simulink model "Quadcopter_Model"  (R2026a)
settings: Solver=FixedStepAuto  StopTime=T  FixedStep=Ts
values from neighbouring files (symbols this model uses):
  a = L/sqrt(2)    [Quadcopter_Commands.m]
  Drag = -0.1    [Quadcopter_Commands.m]
  g = 9.81    [Quadcopter_Commands.m]
  Hover_FeedForward = sqrt((M*g)/(4*Kf))    [Quadcopter_Commands.m]
  Ix = 6*10^(-5)    (= 6e-05)    [Quadcopter_Commands.m]
  Iy = 6*10^(-5)    (= 6e-05)    [Quadcopter_Commands.m]
  Iz = 1.2*10^(-4)    (= 0.00012)    [Quadcopter_Commands.m]
  Kf = 3*10^(-7)    (= 3e-07)    [Quadcopter_Commands.m]
  Km = 3*10^(-9)    (= 3e-09)    [Quadcopter_Commands.m]
  M = 0.07    [Quadcopter_Commands.m]
  Ts = 0.001    [Quadcopter_Commands.m]
undefined symbols (not defined in the file or in its folder): dspblkCoreblockFVToolHelper, gcbh
libraries: simulink x9, matrix_library x5
settings Model: Creator=marco91  LastModifiedBy=marco91
settings OptimizationCC: DefaultUnderspecifiedDataType=single  OptimizeBlockIOStorage=off  BufferReuse=off  OptimizeDataStoreBuffers=off  BusAssignmentInplaceUpdate=off
settings DebuggingCC: ParamPrecisionLossAbsoluteDiffThreshold=0  ParamPrecisionLossRelativeDiffThreshold=0
settings RTWCC: GenCodeOnly=on  GenerateReport=on  BuildConfiguration=Debug  LaunchReport=on
settings CodeAppCC: MATLABSourceComments=on  EnableCustomComments=on
settings GRTTargetCC: MultiInstanceErrorCode=Warning  CombineSignalStateStructs=on  SupportVariableSizeSignals=on

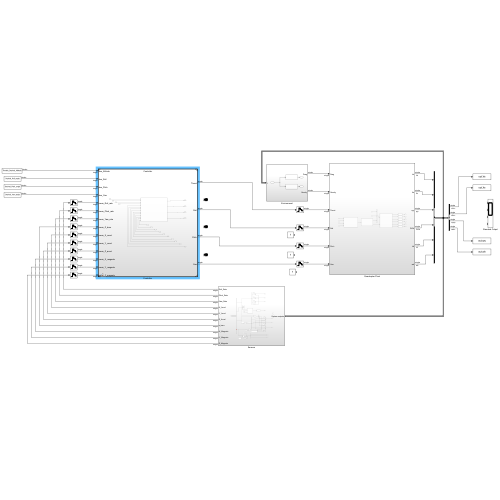
[thumbnail: Simulink's stored preview of the top-level diagram]
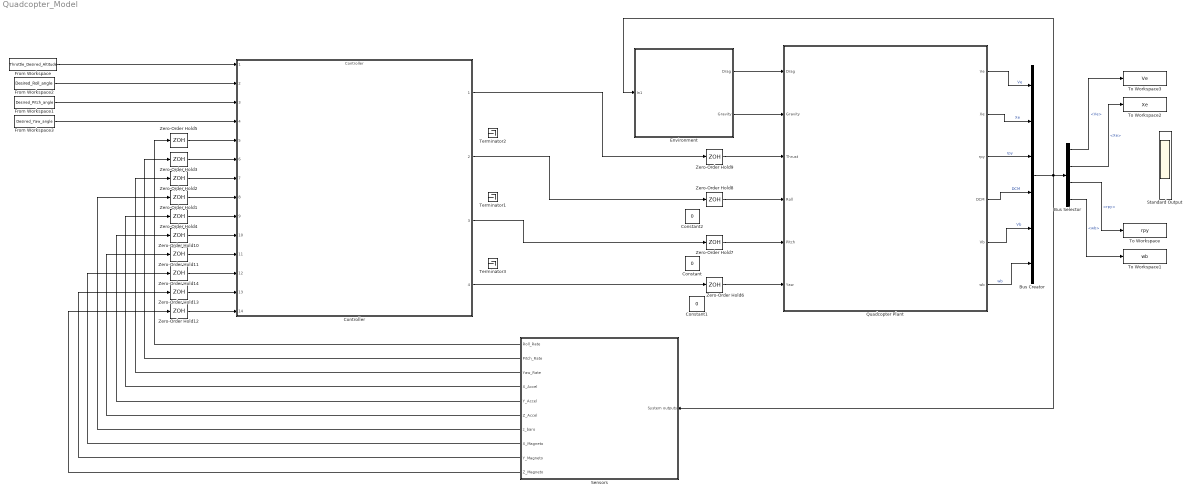
== system Quadcopter_Model ==
  Bus Creator : BusCreator  Inputs=6
  Bus Selector : BusSelector  OutputSignals=Ve,Xe,rpy,wb
  Constant : Constant  Value=0  OutDataTypeStr=single
  Constant1 : Constant  Value=0  OutDataTypeStr=single
  Constant2 : Constant  Value=0  OutDataTypeStr=single
  Controller : ModelReference  ModelNameDialog=Controller  SimulationMode=Normal  ModelReferenceVersion=2.455
  Environment : Subsystem
  From Workspace : FromWorkspace  VariableName=Throttle_Desired_Altitude  SampleTime=Ts
  From Workspace1 : FromWorkspace  VariableName=Desired_Pitch_angle  SampleTime=Ts
  From Workspace2 : FromWorkspace  VariableName=Desired_Roll_angle  SampleTime=Ts
  From Workspace3 : FromWorkspace  VariableName=Desired_Yaw_angle  SampleTime=Ts
  Quadcopter Plant : Subsystem
  Sensors : Subsystem
  Standard Output : Scope  NumInputPorts=4
      settings: ActiveDisplayYMinimum=-2.7234359681606293  ActiveDisplayYMaximum=4.365431159734726
  Terminator1 : Terminator
  Terminator2 : Terminator
  Terminator3 : Terminator
  To Workspace : ToWorkspace  VariableName=rpy  SaveFormat=Timeseries  SampleTime=Ts
  To Workspace1 : ToWorkspace  VariableName=wb  SaveFormat=Timeseries  SampleTime=Ts
  To Workspace2 : ToWorkspace  VariableName=Xe  SaveFormat=Timeseries  SampleTime=Ts
  To Workspace3 : ToWorkspace  VariableName=Ve  SaveFormat=Timeseries  SampleTime=Ts
  Zero-Order Hold1 : ZeroOrderHold  SampleTime=50*Ts
  Zero-Order Hold{2..5,10..11} (6 alike) : ZeroOrderHold  SampleTime=2*Ts
  Zero-Order Hold12 : ZeroOrderHold  SampleTime=10*Ts
  Zero-Order Hold13 : ZeroOrderHold  SampleTime=10*Ts
  Zero-Order Hold14 : ZeroOrderHold  SampleTime=10*Ts
  Zero-Order Hold{6..9} (4 alike) : ZeroOrderHold  SampleTime=Ts
  wires:
  Bus Creator/1 -> Environment/1(In1), Bus Selector/1, Sensors/1(System outputs)
  Bus Selector/1 -> To Workspace3/1  "<Ve>"
  Bus Selector/2 -> To Workspace2/1  "<Xe>"
  Bus Selector/3 -> To Workspace/1  "<rpy>"
  Bus Selector/4 -> To Workspace1/1  "<wb>"
  Quadcopter Plant/1(Ve) -> Bus Creator/1  "Ve"
  Quadcopter Plant/2(Xe) -> Bus Creator/2  "Xe"
  Quadcopter Plant/3(rpy) -> Bus Creator/3  "rpy"
  Quadcopter Plant/4(DCM) -> Bus Creator/4  "DCM"
  Quadcopter Plant/5(Vb) -> Bus Creator/5  "Vb"
  Quadcopter Plant/6(wb) -> Bus Creator/6  "wb"
  From Workspace/1 -> Controller/1
  From Workspace2/1 -> Controller/2
  From Workspace1/1 -> Controller/3
  From Workspace3/1 -> Controller/4
  Zero-Order Hold4/1 -> Controller/9
  Zero-Order Hold5/1 -> Controller/5
  Zero-Order Hold3/1 -> Controller/6
  Zero-Order Hold2/1 -> Controller/7
  Zero-Order Hold1/1 -> Controller/8
  Sensors/1(Roll_Rate) -> Zero-Order Hold5/1
  Sensors/2(Pitch_Rate) -> Zero-Order Hold3/1
  Sensors/3(Yaw_Rate) -> Zero-Order Hold2/1
  Sensors/4(X_Accel) -> Zero-Order Hold4/1
  Sensors/5(Y_Accel) -> Zero-Order Hold10/1
  Sensors/6(Z_Accel) -> Zero-Order Hold11/1
  Zero-Order Hold10/1 -> Controller/10
  Zero-Order Hold11/1 -> Controller/11
  Zero-Order Hold12/1 -> Controller/14
  Zero-Order Hold13/1 -> Controller/13
  Zero-Order Hold14/1 -> Controller/12
  Sensors/7(z_baro) -> Zero-Order Hold1/1
  Sensors/8(X_Magneto) -> Zero-Order Hold14/1
  Sensors/9(Y_Magneto) -> Zero-Order Hold13/1
  Sensors/10(Z_Magneto) -> Zero-Order Hold12/1
  Environment/1(Drag) -> Quadcopter Plant/1(Drag)
  Environment/2(Gravity) -> Quadcopter Plant/2(Gravity)
  Zero-Order Hold9/1 -> Quadcopter Plant/3(Thrust)
  Controller/1 -> Zero-Order Hold9/1
  Zero-Order Hold6/1 -> Quadcopter Plant/6(Yaw)
  Controller/4 -> Zero-Order Hold6/1
  Zero-Order Hold7/1 -> Quadcopter Plant/5(Pitch)
  Zero-Order Hold8/1 -> Quadcopter Plant/4(Roll)
  Controller/3 -> Zero-Order Hold7/1
  Controller/2 -> Zero-Order Hold8/1

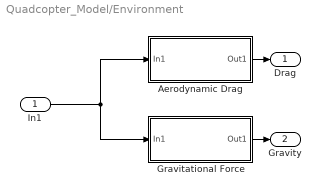
== system Quadcopter_Model/Environment ==
  In1 : Inport  OutDataTypeStr=single
  Aerodynamic Drag : Subsystem
  Gravitational Force : Subsystem
  Drag : Outport
  Gravity : Outport  Port=2
  wires:
  Gravitational Force/1(Out1) -> Gravity/1
  Aerodynamic Drag/1(Out1) -> Drag/1
  In1/1 -> Gravitational Force/1(In1), Aerodynamic Drag/1(In1)

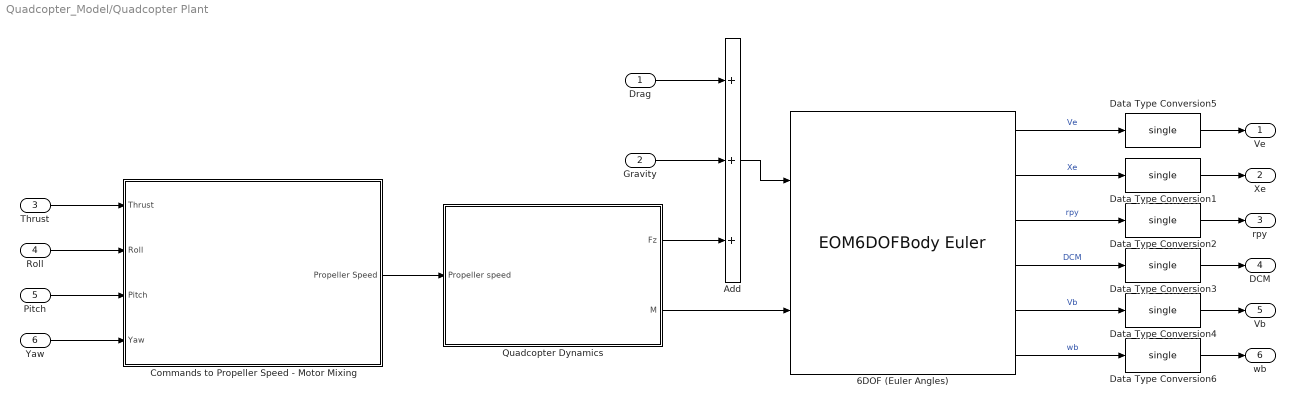
== system Quadcopter_Model/Quadcopter Plant ==
  Drag : Inport  OutDataTypeStr=single
  Gravity : Inport  Port=2  OutDataTypeStr=single
  Thrust : Inport  Port=3  OutDataTypeStr=single
  Roll : Inport  Port=4  OutDataTypeStr=single
  Pitch : Inport  Port=5  OutDataTypeStr=single
  Yaw : Inport  Port=6  OutDataTypeStr=single
  6DOF (Euler Angles) : EOM6DOFBodyEuler  mass_0=M  inertia=[Ix, 0, 0; 0, Iy, 0; 0, 0, Iz]
  Add : Sum  Inputs=+++  OutDataTypeStr=double
  "Commands to Propeller Speed - Motor Mixing " : Subsystem
  Data Type Conversion{1..6} (6 alike) : DataTypeConversion  OutDataTypeStr=single  SaturateOnIntegerOverflow=off  RndMeth=Floor
  Quadcopter Dynamics : Subsystem
  Ve : Outport  OutDataTypeStr=single
  Xe : Outport  Port=2  OutDataTypeStr=single
  rpy : Outport  Port=3  OutDataTypeStr=single
  DCM : Outport  Port=4  OutDataTypeStr=single
  Vb : Outport  Port=5  OutDataTypeStr=single
  wb : Outport  Port=6  OutDataTypeStr=single
  wires:
  "Commands to Propeller Speed - Motor Mixing "/1(Propeller Speed) -> Quadcopter Dynamics/1(Propeller speed)
  Quadcopter Dynamics/1(Fz) -> Add/3
  Quadcopter Dynamics/2(M) -> 6DOF (Euler Angles)/2
  6DOF (Euler Angles)/2 -> Data Type Conversion1/1  "Xe"
  Pitch/1 -> "Commands to Propeller Speed - Motor Mixing "/3(Pitch)
  Add/1 -> 6DOF (Euler Angles)/1
  6DOF (Euler Angles)/5 -> Data Type Conversion4/1  "Vb"
  Thrust/1 -> "Commands to Propeller Speed - Motor Mixing "/1(Thrust)
  6DOF (Euler Angles)/3 -> Data Type Conversion2/1  "rpy"
  6DOF (Euler Angles)/4 -> Data Type Conversion3/1  "DCM"
  Gravity/1 -> Add/2
  6DOF (Euler Angles)/1 -> Data Type Conversion5/1  "Ve"
  6DOF (Euler Angles)/6 -> Data Type Conversion6/1  "wb"
  Drag/1 -> Add/1
  Yaw/1 -> "Commands to Propeller Speed - Motor Mixing "/4(Yaw)
  Roll/1 -> "Commands to Propeller Speed - Motor Mixing "/2(Roll)
  Data Type Conversion6/1 -> wb/1
  Data Type Conversion4/1 -> Vb/1
  Data Type Conversion3/1 -> DCM/1
  Data Type Conversion2/1 -> rpy/1
  Data Type Conversion1/1 -> Xe/1
  Data Type Conversion5/1 -> Ve/1

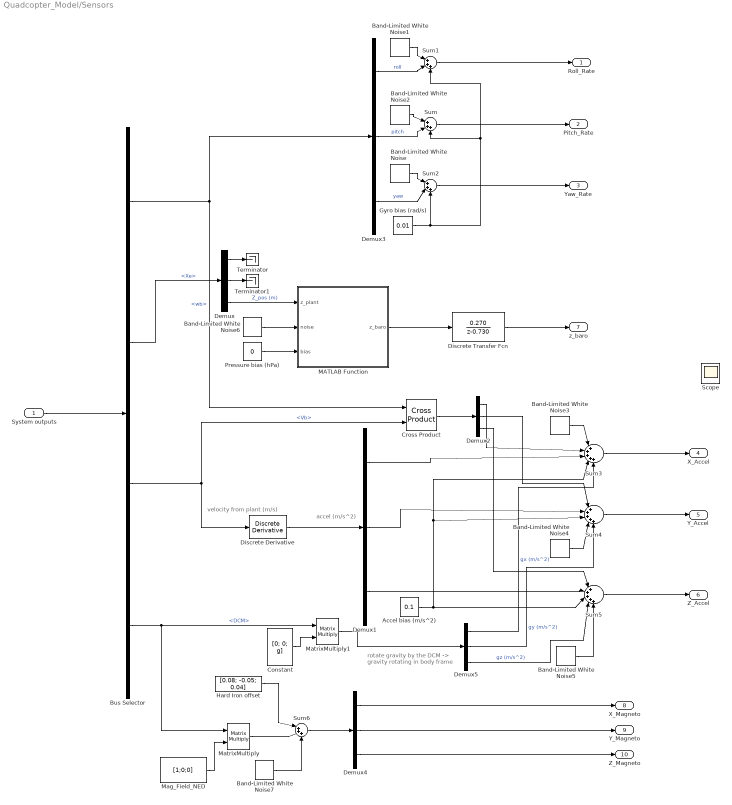
== system Quadcopter_Model/Sensors ==
  note: rotate gravity by the DCM
      | -> gravity rotating in body frame
  note: accel (m/s^2)
  note: velocity from
      | plant (m/s)
  System outputs : Inport
  Accel bias (m/s^2) : Constant  Value=0.1  OutDataTypeStr=single
  Band-Limited White Noise : simulink/Sources/Band-Limited White Noise  Cov=4e-9  Ts=Ts  seed=[23341]
  Band-Limited White Noise1 : simulink/Sources/Band-Limited White Noise  Cov=4e-9  Ts=Ts  seed=[23342]
  Band-Limited White Noise2 : simulink/Sources/Band-Limited White Noise  Cov=4e-9  Ts=Ts  seed=[23343]
  Band-Limited White Noise3 : simulink/Sources/Band-Limited White Noise  Cov=4e-7  Ts=Ts  seed=[23342]
  Band-Limited White Noise4 : simulink/Sources/Band-Limited White Noise  Cov=4e-7  Ts=Ts  seed=[23343]
  Band-Limited White Noise5 : simulink/Sources/Band-Limited White Noise  Cov=4e-7  Ts=Ts  seed=[23341]
  Band-Limited White Noise6 : simulink/Sources/Band-Limited White Noise  Cov=4e-7  Ts=Ts  seed=[23341]
  Band-Limited White Noise7 : simulink/Sources/Band-Limited White Noise  Cov=4e-7  Ts=Ts  seed=[23341]
  Bus Selector : BusSelector  OutputSignals=wb,Xe,Vb,DCM
  Constant : Constant  Value=[0; 0; g]  VectorParams1D=off
  Cross Product : matrix_library/Cross Product
  Demux{,1..5} (6 alike) : Demux  Outputs=3
  Discrete Transfer Fcn : DiscreteTransferFcn  LoadFcn=dspblkCoreblockFVToolHelper(gcbh,'load');  Numerator=[0.270]  Denominator="[1  -0.730]"
      settings: CopyFcn=dspblkCoreblockFVToolHelper(gcbh,'copy');  DeleteFcn=dspblkCoreblockFVToolHelper(gcbh,'close');  ModelCloseFcn=dspblkCoreblockFVToolHelper(gcbh,'close');  PreSaveFcn=dspblkCoreblockFVToolHelper(gcbh,'presave');  PostSaveFcn=dspblkCoreblockFVToolHelper(gcbh,'postsave');  CloseFcn=dspblkCoreblockFVToolHelper(gcbh,'close');
  Discrete Derivative : simulink/Discrete/Discrete Derivative  gainval=1.0  ICPrevScaledInput=0.0  OutMin=[]  OutMax=[]  OutDataTypeStr=single  OutputDataTypeScalingMode=single  OutDataType=fixdt(1, 16)  OutScaling=2^-10  DoSatur=off
  Gyro bias (rad/s) : Constant  Value=0.01  OutDataTypeStr=single
  Hard Iron offset : Constant  Value=[0.08; -0.05; 0.04]  VectorParams1D=off  OutDataTypeStr=single
  MATLAB Function : MATLAB Function  TreatAsAtomicUnit=on
  Mag_Field_NED : Constant  Value=[1;0;0]  VectorParams1D=off
  MatrixMultiply : Product  Multiplication=Matrix(*)
  MatrixMultiply1 : Product  Multiplication=Matrix(*)
  Pressure bias (hPa) : Constant  Value=0  OutDataTypeStr=single
  Scope : Scope
      settings: ActiveDisplayYMinimum=-1  ActiveDisplayYMaximum=1
  Sum{,1..2,6} (4 alike) : Sum  Inputs=|+++  OutDataTypeStr=single
  Sum3 : Sum  Inputs=|+++++  OutDataTypeStr=single
  Sum4 : Sum  Inputs=|+++++  OutDataTypeStr=single
  Sum5 : Sum  Inputs=|+++++  OutDataTypeStr=single
  Terminator : Terminator
  Terminator1 : Terminator
  Roll_Rate : Outport  OutDataTypeStr=single
  Pitch_Rate : Outport  Port=2  OutDataTypeStr=single
  Yaw_Rate : Outport  Port=3  OutDataTypeStr=single
  X_Accel : Outport  Port=4  OutDataTypeStr=single
  Y_Accel : Outport  Port=5  OutDataTypeStr=single
  Z_Accel : Outport  Port=6  OutDataTypeStr=single
  z_baro : Outport  Port=7  OutDataTypeStr=single
  X_Magneto : Outport  Port=8  OutDataTypeStr=single
  Y_Magneto : Outport  Port=9  OutDataTypeStr=single
  Z_Magneto : Outport  Port=10  OutDataTypeStr=single
  wires:
  System outputs/1 -> Bus Selector/1
  Bus Selector/1 -> Cross Product/1, Demux3/1  "<wb>"
  Sum2/1 -> Yaw_Rate/1
  Sum1/1 -> Roll_Rate/1
  Sum/1 -> Pitch_Rate/1
  Demux3/1 -> Sum1/2  "roll"
  Band-Limited White Noise1/1 -> Sum1/1
  Demux3/3 -> Sum2/2  "yaw"
  Demux3/2 -> Sum/2  "pitch"
  Band-Limited White Noise2/1 -> Sum/1
  Band-Limited White Noise/1 -> Sum2/1
  Gyro bias (rad/s)/1 -> Sum1/3, Sum/3, Sum2/3
  Demux1/1 -> Sum3/3
  Demux1/2 -> Sum4/2
  Demux1/3 -> Sum5/2
  Band-Limited White Noise3/1 -> Sum3/1
  Accel bias (m/s^2)/1 -> Sum3/4, Sum4/3, Sum5/3
  Sum4/1 -> Y_Accel/1
  Sum3/1 -> X_Accel/1
  Bus Selector/2 -> Demux/1  "<Xe>"
  Demux/1 -> Terminator/1
  Demux/2 -> Terminator1/1
  Bus Selector/3 -> Discrete Derivative/1, Cross Product/2  "<Vb>"
  Cross Product/1 -> Demux2/1
  Demux2/3 -> Sum5/1
  Demux2/1 -> Sum3/2
  Band-Limited White Noise5/1 -> Sum5/5
  Band-Limited White Noise4/1 -> Sum4/4
  Demux2/2 -> Sum4/1
  Demux/3 -> MATLAB Function/1(z_plant)  "Z_pos (m)"
  Pressure bias (hPa)/1 -> MATLAB Function/3(bias)
  Band-Limited White Noise6/1 -> MATLAB Function/2(noise)
  Mag_Field_NED/1 -> MatrixMultiply/2
  Bus Selector/4 -> MatrixMultiply/1, MatrixMultiply1/1  "<DCM>"
  MatrixMultiply/1 -> Sum6/2
  Band-Limited White Noise7/1 -> Sum6/3
  Hard Iron offset/1 -> Sum6/1
  Sum6/1 -> Demux4/1
  Demux4/1 -> X_Magneto/1
  Demux4/2 -> Y_Magneto/1
  Demux4/3 -> Z_Magneto/1
  Discrete Derivative/1 -> Demux1/1
  Sum5/1 -> Z_Accel/1
  MATLAB Function/1(z_baro) -> Discrete Transfer Fcn/1
  Discrete Transfer Fcn/1 -> z_baro/1
  MatrixMultiply1/1 -> Demux5/1
  Demux5/1 -> Sum3/5  "gx (m/s^2)"
  Demux5/3 -> Sum5/4  "gz (m/s^2)"
  Demux5/2 -> Sum4/5  "gy (m/s^2)"
  Constant/1 -> MatrixMultiply1/2

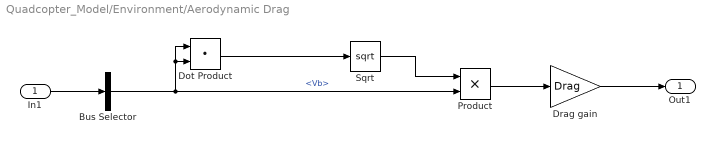
== system Quadcopter_Model/Environment/Aerodynamic Drag ==
  In1 : Inport  OutDataTypeStr=single
  Bus Selector : BusSelector  OutputSignals=Vb
  Dot Product : DotProduct  OutDataTypeStr=single
  Drag gain : Gain  Gain=Drag  OutDataTypeStr=single
  Product : Product  OutDataTypeStr=single
  Sqrt : Sqrt  OutDataTypeStr=single  IntermediateResultsDataTypeStr=single
  Out1 : Outport
  wires:
  Drag gain/1 -> Out1/1
  Product/1 -> Drag gain/1
  Sqrt/1 -> Product/1
  Bus Selector/1 -> Dot Product/1, Dot Product/2, Product/2  "<Vb>"
  In1/1 -> Bus Selector/1
  Dot Product/1 -> Sqrt/1

== system Quadcopter_Model/Environment/Gravitational Force ==
  note: (Gravitational) Force given by the gravitational acceleration multiplied by the mass
  In1 : Inport  OutDataTypeStr=single
  Gravitational Acceleration : Subsystem
  Mass [Kg] : Gain  Gain=M
  Out1 : Outport
  wires:
  In1/1 -> Gravitational Acceleration/1(In1)
  Gravitational Acceleration/1(Out1) -> Mass [Kg]/1
  Mass [Kg]/1 -> Out1/1

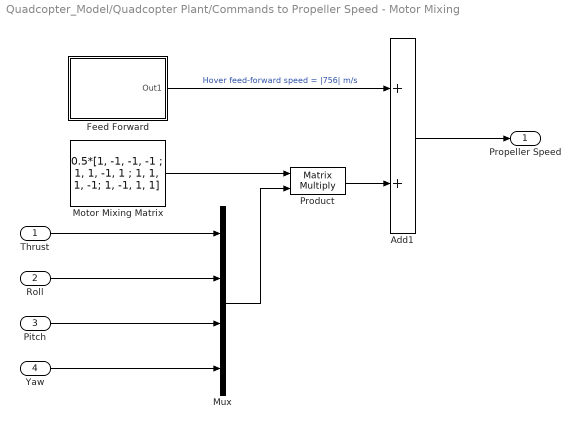
== system Quadcopter_Model/Quadcopter Plant/Commands to Propeller Speed - Motor Mixing  ==
  Thrust : Inport
  Roll : Inport  Port=2  OutDataTypeStr=single
  Pitch : Inport  Port=3  OutDataTypeStr=single
  Yaw : Inport  Port=4  OutDataTypeStr=single
  Add1 : Sum
  Feed Forward : Subsystem
  Motor Mixing Matrix : Constant  Value="0.5*[1, -1, -1, -1 ; 1, 1, -1, 1 ;   1, 1, 1, -1;  1, -1, 1, 1]"  VectorParams1D=off  OutDataTypeStr=single
  Mux : Mux
  Product : Product  Multiplication=Matrix(*)  OutDataTypeStr=single
  Propeller Speed : Outport  OutDataTypeStr=single
  wires:
  Feed Forward/1(Out1) -> Add1/1  "Hover feed-forward speed = |756| m/s"
  Mux/1 -> Product/2
  Pitch/1 -> Mux/3
  Product/1 -> Add1/2
  Roll/1 -> Mux/2
  Motor Mixing Matrix/1 -> Product/1
  Yaw/1 -> Mux/4
  Add1/1 -> Propeller Speed/1
  Thrust/1 -> Mux/1

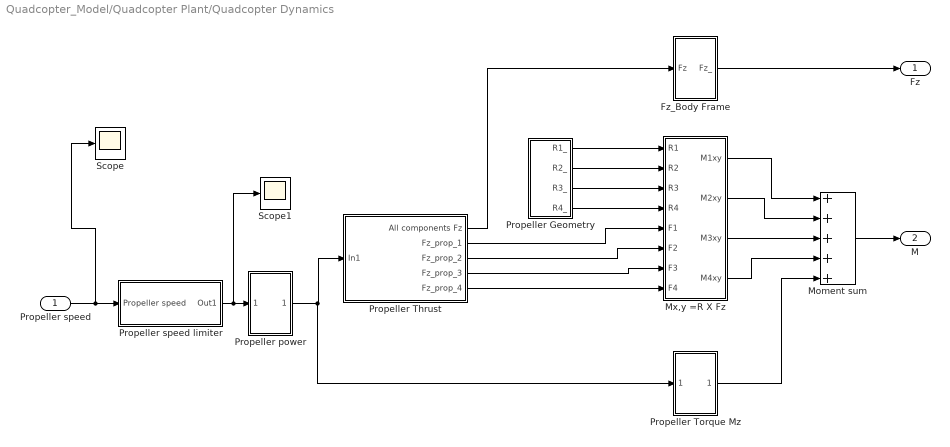
== system Quadcopter_Model/Quadcopter Plant/Quadcopter Dynamics ==
  Propeller speed : Inport  OutDataTypeStr=single
  Fz_Body Frame : Subsystem
  Moment sum : Sum  Inputs=+++++  OutDataTypeStr=double
  Mx,y =R X Fz : Subsystem
  Propeller Geometry : Subsystem
  Propeller Thrust : Subsystem
  Propeller Torque Mz : Subsystem
  Propeller power : Subsystem
  Propeller speed limiter : Subsystem
  Scope : Scope
      settings: ActiveDisplayYMinimum=-967.50824737548828  ActiveDisplayYMaximum=-720.62401580810547  DataLoggingVariableName=ScopeData4
  Scope1 : Scope
      settings: ActiveDisplayYMinimum=-967.50824737548828  ActiveDisplayYMaximum=-720.62401580810547  DataLoggingVariableName=ScopeData2
  Fz : Outport  OutDataTypeStr=single
  M : Outport  Port=2  OutDataTypeStr=double
  wires:
  Propeller speed/1 -> Scope/1, Propeller speed limiter/1(Propeller speed)
  Propeller speed limiter/1(Out1) -> Scope1/1, Propeller power/1(In1)
  Propeller power/1(Out1) -> Propeller Torque Mz/1(In1), Propeller Thrust/1(In1)
  Propeller Thrust/1(All components Fz) -> Fz_Body Frame/1(Fz)
  Propeller Thrust/2(Fz_prop_1) -> Mx,y =R X Fz/5(F1)
  Propeller Thrust/3(Fz_prop_2) -> Mx,y =R X Fz/6(F2)
  Propeller Thrust/4(Fz_prop_3) -> Mx,y =R X Fz/7(F3)
  Propeller Thrust/5(Fz_prop_4) -> Mx,y =R X Fz/8(F4)
  Propeller Geometry/4(R4_) -> Mx,y =R X Fz/4(R4)
  Propeller Geometry/3(R3_) -> Mx,y =R X Fz/3(R3)
  Propeller Geometry/2(R2_) -> Mx,y =R X Fz/2(R2)
  Propeller Geometry/1(R1_) -> Mx,y =R X Fz/1(R1)
  Fz_Body Frame/1(Fz_) -> Fz/1
  Moment sum/1 -> M/1
  Mx,y =R X Fz/1(M1xy) -> Moment sum/1
  Mx,y =R X Fz/2(M2xy) -> Moment sum/2
  Mx,y =R X Fz/3(M3xy) -> Moment sum/3
  Mx,y =R X Fz/4(M4xy) -> Moment sum/4
  Propeller Torque Mz/1(Out1) -> Moment sum/5

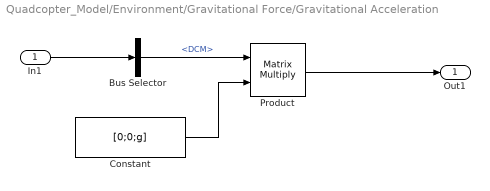
== system Quadcopter_Model/Environment/Gravitational Force/Gravitational Acceleration ==
  In1 : Inport  OutDataTypeStr=single
  Bus Selector : BusSelector  OutputSignals=DCM
  Constant : Constant  Value=[0;0;g]  OutDataTypeStr=single
  Product : Product  Multiplication=Matrix(*)  OutDataTypeStr=single
  Out1 : Outport  OutDataTypeStr=single
  wires:
  Constant/1 -> Product/2
  In1/1 -> Bus Selector/1
  Bus Selector/1 -> Product/1  "<DCM>"
  Product/1 -> Out1/1

== system Quadcopter_Model/Quadcopter Plant/Commands to Propeller Speed - Motor Mixing /Feed Forward ==
  Constant1 : Constant  Value=[1;1;1;1]  OutDataTypeStr=single
  Direction : Gain  Gain=-1  OutDataTypeStr=single
  Hover feedforward : Gain  Gain=Hover_FeedForward  OutDataTypeStr=single
  Out1 : Outport  OutDataTypeStr=single
  wires:
  Direction/1 -> Hover feedforward/1
  Constant1/1 -> Direction/1
  Hover feedforward/1 -> Out1/1

== system Quadcopter_Model/Quadcopter Plant/Quadcopter Dynamics/Fz_Body Frame ==
  Fz : Inport
  Sum of Elements : Sum  Inputs=+
  "z-vector " : Subsystem
  Fz_ : Outport
  wires:
  Sum of Elements/1 -> "z-vector "/1(Fz_in)
  "z-vector "/1(Fz_out) -> Fz_/1
  Fz/1 -> Sum of Elements/1

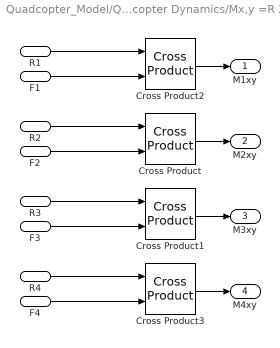
== system Quadcopter_Model/Quadcopter Plant/Quadcopter Dynamics/Mx,y =R X Fz ==
  R1 : Inport
  R2 : Inport  Port=2
  R3 : Inport  Port=3
  R4 : Inport  Port=4
  F1 : Inport  Port=5
  F2 : Inport  Port=6
  F3 : Inport  Port=7
  F4 : Inport  Port=8
  Cross Product{,1..3} (4 alike) : matrix_library/Cross Product
  M1xy : Outport
  M2xy : Outport  Port=2
  M3xy : Outport  Port=3
  M4xy : Outport  Port=4
  wires:
  F4/1 -> Cross Product3/2
  Cross Product/1 -> M2xy/1
  Cross Product2/1 -> M1xy/1
  F1/1 -> Cross Product2/2
  R2/1 -> Cross Product/1
  F3/1 -> Cross Product1/2
  Cross Product3/1 -> M4xy/1
  Cross Product1/1 -> M3xy/1
  F2/1 -> Cross Product/2
  R3/1 -> Cross Product1/1
  R1/1 -> Cross Product2/1
  R4/1 -> Cross Product3/1

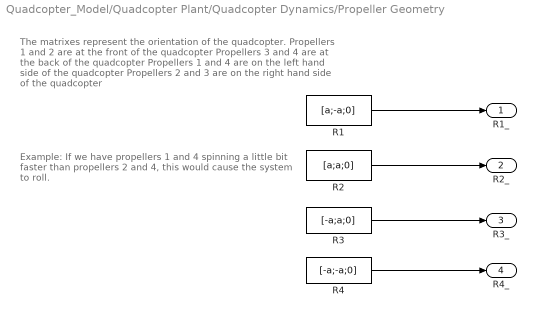
== system Quadcopter_Model/Quadcopter Plant/Quadcopter Dynamics/Propeller Geometry ==
  note: Example:
      | If we have propellers 1 and 4 spinning a little bit faster
      | than propellers 2 and 4, this would cause the system
      | to roll.
  note: The matrixes represent the orientation of the quadcopter.
      | Propellers 1 and 2 are at the front of the quadcopter
      | Propellers 3 and 4 are at the back of the quadcopter
      | Propellers 1 and 4 are on the left hand side of the quadcopter
      | Propellers 2 and 3 are on the right hand side of the quadcopter
  R1 : Constant  Value=[a;-a;0]
  R2 : Constant  Value=[a;a;0]
  R3 : Constant  Value=[-a;a;0]
  R4 : Constant  Value=[-a;-a;0]
  R1_ : Outport
  R2_ : Outport  Port=2
  R3_ : Outport  Port=3
  R4_ : Outport  Port=4
  wires:
  R1/1 -> R1_/1
  R4/1 -> R4_/1
  R3/1 -> R3_/1
  R2/1 -> R2_/1

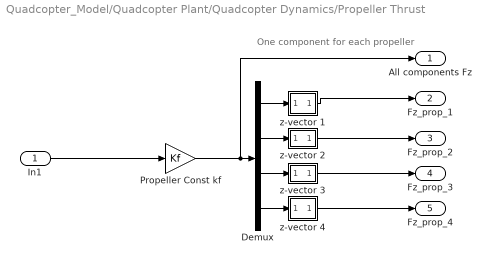
== system Quadcopter_Model/Quadcopter Plant/Quadcopter Dynamics/Propeller Thrust ==
  note: One component for each propeller
  In1 : Inport
  Demux : Demux
  Propeller Const kf : Gain  Gain=Kf
  z-vector 1 : Subsystem
  z-vector 2 : Subsystem
  z-vector 3 : Subsystem
  z-vector 4 : Subsystem
  All components Fz : Outport
  Fz_prop_1 : Outport  Port=2
  Fz_prop_2 : Outport  Port=3
  Fz_prop_3 : Outport  Port=4
  Fz_prop_4 : Outport  Port=5
  wires:
  Demux/4 -> z-vector 4/1(In1)
  Demux/1 -> z-vector 1/1(In1)
  z-vector 3/1(Out1) -> Fz_prop_3/1
  z-vector 2/1(Out1) -> Fz_prop_2/1
  Propeller Const kf/1 -> All components Fz/1, Demux/1
  z-vector 1/1(Out1) -> Fz_prop_1/1
  Demux/2 -> z-vector 2/1(In1)
  Demux/3 -> z-vector 3/1(In1)
  z-vector 4/1(Out1) -> Fz_prop_4/1
  In1/1 -> Propeller Const kf/1

== system Quadcopter_Model/Quadcopter Plant/Quadcopter Dynamics/Propeller Torque Mz ==
  In1 : Inport  OutDataTypeStr=single
  Motor Torq Const km : Gain  Gain=Km  OutDataTypeStr=single
  z-torque : Subsystem
  z-vector 5 : Subsystem
  Out1 : Outport  OutDataTypeStr=single
  wires:
  z-torque/1(Out1) -> z-vector 5/1(In1)
  Motor Torq Const km/1 -> z-torque/1(In1)
  z-vector 5/1(Out1) -> Out1/1
  In1/1 -> Motor Torq Const km/1

== system Quadcopter_Model/Quadcopter Plant/Quadcopter Dynamics/Propeller power ==
  In1 : Inport
  Abs : Abs  SaturateOnIntegerOverflow=off
  Product : Product
  Out1 : Outport
  wires:
  In1/1 -> Product/2, Abs/1
  Abs/1 -> Product/1
  Product/1 -> Out1/1

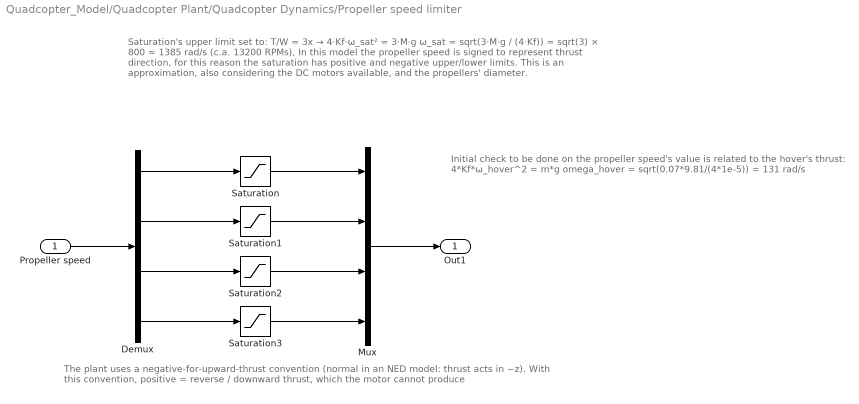
== system Quadcopter_Model/Quadcopter Plant/Quadcopter Dynamics/Propeller speed limiter ==
  note: The plant uses a negative-for-upward-thrust convention (normal in an NED model: thrust acts in −z).
      | With this convention, positive = reverse / downward thrust, which the motor cannot produce
  note: Initial check to be done on the propeller speed's value is related to the hover's thrust:
      | 4*Kf*​ω_hover^2 ​= m*g
      | omega_hover = sqrt(0.07*9.81/(4*1e-5)) = 131 rad/s
  note: Saturation's upper limit set to:
      | T/W = 3x → 4·Kf·ω_sat² = 3·M·g ω_sat = sqrt(3·M·g / (4·Kf)) = sqrt(3) × 800 ≈ 1385 rad/s (c.a. 13200 RPMs),
      | In this model the propeller speed is signed to represent thrust direction, for this reason
      | the saturation has positive and negative upper/lower limits.
      | This is an approximation, also considering the DC motors available, and the propellers' diameter.
  Propeller speed : Inport  OutDataTypeStr=single
  Demux : Demux
  Mux : Mux
  Saturation{,1..3} (4 alike) : Saturate  UpperLimit=0  LowerLimit=-1400
  Out1 : Outport
  wires:
  Mux/1 -> Out1/1
  Demux/4 -> Saturation3/1
  Demux/3 -> Saturation2/1
  Demux/2 -> Saturation1/1
  Propeller speed/1 -> Demux/1
  Demux/1 -> Saturation/1
  Saturation/1 -> Mux/1
  Saturation1/1 -> Mux/2
  Saturation2/1 -> Mux/3
  Saturation3/1 -> Mux/4

== system Quadcopter_Model/Quadcopter Plant/Quadcopter Dynamics/Fz_Body Frame/z-vector  ==
  Fz_in : Inport
  Divide : Product  Inputs=**
  az : Constant  Value=[0;0;1]  OutDataTypeStr=single
  Fz_out : Outport
  wires:
  az/1 -> Divide/1
  Divide/1 -> Fz_out/1
  Fz_in/1 -> Divide/2

== system Quadcopter_Model/Quadcopter Plant/Quadcopter Dynamics/Propeller Thrust/z-vector 1 ==
  In1 : Inport
  Divide : Product  Inputs=**
  z_axis : Constant  Value=[0;0;1]
  Out1 : Outport
  wires:
  z_axis/1 -> Divide/1
  Divide/1 -> Out1/1
  In1/1 -> Divide/2

== system Quadcopter_Model/Quadcopter Plant/Quadcopter Dynamics/Propeller Thrust/z-vector 2 ==
  In1 : Inport
  Divide : Product  Inputs=**
  az : Constant  Value=[0;0;1]
  Out1 : Outport
  wires:
  az/1 -> Divide/1
  Divide/1 -> Out1/1
  In1/1 -> Divide/2

== system Quadcopter_Model/Quadcopter Plant/Quadcopter Dynamics/Propeller Thrust/z-vector 3 ==
  In1 : Inport
  Divide : Product  Inputs=**
  az : Constant  Value=[0;0;1]
  Out1 : Outport
  wires:
  az/1 -> Divide/1
  Divide/1 -> Out1/1
  In1/1 -> Divide/2

== system Quadcopter_Model/Quadcopter Plant/Quadcopter Dynamics/Propeller Thrust/z-vector 4 ==
  In1 : Inport
  Divide : Product  Inputs=**
  az : Constant  Value=[0;0;1]
  Out1 : Outport
  wires:
  az/1 -> Divide/1
  Divide/1 -> Out1/1
  In1/1 -> Divide/2

== system Quadcopter_Model/Quadcopter Plant/Quadcopter Dynamics/Propeller Torque Mz/z-torque ==
  In1 : Inport
  Constant : Constant  Value=[-1; 1; -1; 1]  OutDataTypeStr=single
  Product1 : Product  OutDataTypeStr=single
  Sum of Elements : Sum  Inputs=+  OutDataTypeStr=single
  Out1 : Outport  OutDataTypeStr=single
  wires:
  Constant/1 -> Product1/1
  In1/1 -> Product1/2
  Product1/1 -> Sum of Elements/1
  Sum of Elements/1 -> Out1/1

== system Quadcopter_Model/Quadcopter Plant/Quadcopter Dynamics/Propeller Torque Mz/z-vector 5 ==
  In1 : Inport  OutDataTypeStr=single
  Divide : Product  Inputs=**  OutDataTypeStr=single
  az : Constant  Value=[0;0;1]  OutDataTypeStr=single
  Out1 : Outport
  wires:
  az/1 -> Divide/1
  Divide/1 -> Out1/1
  In1/1 -> Divide/2

== matlab function Quadcopter_Model/Sensors/MATLAB Function ==
  data: z_plant input; z_baro output; noise input; bias input
function z_baro = BarometerModel(z_plant, noise, bias)

% Model convention: z = -1 means 1 m above reference
h  = -z_plant; % Initial positive upwards altitude (m)

P0 = single(1013.25);      % Sea level pressure (hPa)
Atm_mul = single(44330.0); % Empirically derived atmospheric multiplier: standardizes how pressure correlate to altitude

% Altitude -> pressure
P = P0 * (single(1.0) - h / Atm_mul)^single(5.255); % (hPa)

% Add pressure sensor noise/bias
P_meas = P + noise + bias;

% Pressure -> altitude
h_baro = Atm_mul * (single(1.0) - (P_meas / P0)^single(1.0/5.255)); % barometric altitude, positive upward

% Convert back to your plant z convention
z_baro = -h_baro; % barometer Z-position measurement in plant coordinates (z-axis sign convention)
